simulink model "GridN3"  (R2021a)
settings: Solver=FixedStepAuto  StartTime=0  StopTime=0.2  FixedStep=0.2  RelTol=1e-3
libraries: spsDistributedParametersLineLib x23, spsThreePhaseSeriesRLCLoadLib x6, spsThreePhaseVIMeasurementLib x2, spsGroundLib x1, spsThreePhaseSourceLib x1, spsSeriesRLCBranchLib x1, spspowerguiLib x1
settings Model: Creator=miair  LastModifiedBy=Admin
settings SolverCC: AlgebraicLoopSolver=TrustRegion
settings DebuggingCC: SFMachineParentedDataDiag=warning  ArithmeticOperatorsInVariantConditions=warning
settings SFSimCC: SimUseLocalCustomCode=off  CustomCodeUndefinedFunction=UseInterfaceOnly
settings RTWCC: RTWUseLocalCustomCode=off
settings CodeAppCC: StateflowObjectComments=on
settings SimscapeCC: SimscapeNormalizeSystem=off

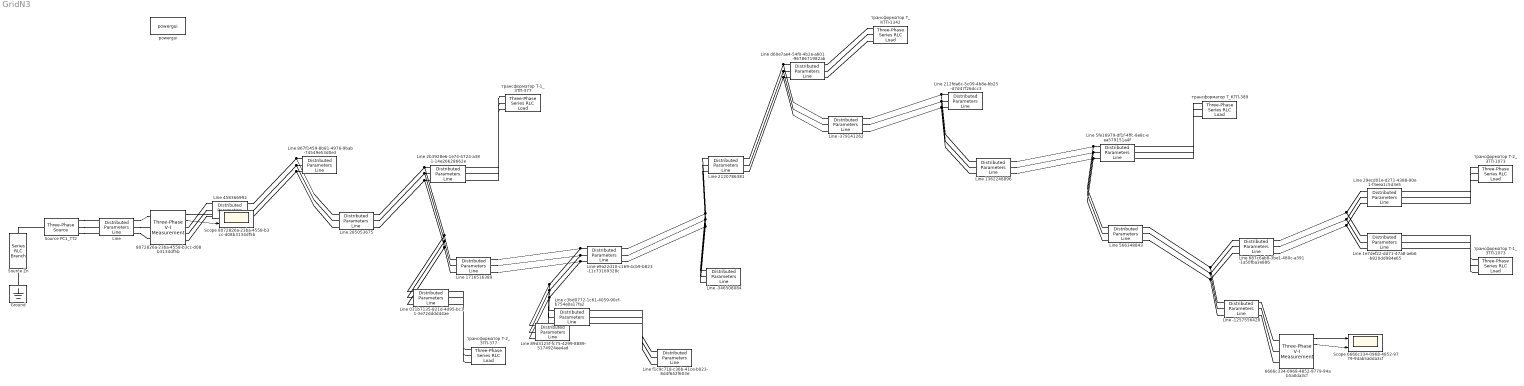
== system GridN3 ==
  6666c334-0968-4852-9779-94ab5a0da3cf : spsThreePhaseVIMeasurementLib/Three-Phase V-I Measurement  VoltageMeasurement=phase-to-ground  SetLabelV=off  LabelV=Vabc  Vpu=off  VpuLL=off  CurrentMeasurement=yes  SetLabelI=off  LabelI=Iabc  Ipu=off  Pbase=100e6  Vbase=500e3  OutputType=Complex  PhasorSimulation=on  PSBequivalent=0
  8072826a-23ba-4558-b3cc-d08b3134df5b : spsThreePhaseVIMeasurementLib/Three-Phase V-I Measurement  VoltageMeasurement=phase-to-ground  SetLabelV=off  LabelV=Vabc  Vpu=off  VpuLL=off  CurrentMeasurement=yes  SetLabelI=off  LabelI=Iabc  Ipu=off  Pbase=100e6  Vbase=500e3  OutputType=Complex  PhasorSimulation=on  PSBequivalent=0
  Ground : spsGroundLib/Ground  LConnTagsString=a
  Line : spsDistributedParametersLineLib/Distributed Parameters Line  Phases=3  Length=0.01  Frequency=50  Resistance=[0.476003738225748 0.351747138225748 0.351747138225748;0.351747138225748 0.476003738225748 0.351747138225748;0.351747138225748 0.351747138225748 0.476003738225748]  Inductance=[0.000705954362986426 0.000459934243504405 0.000459934243504405;0.000459934243504405 0.000705954362986426 0.000459934243504405;0.000459934243504405 0.000459934243504405 0.000705954362986426]  Capacitance=[5.7561313269996e-07 -1.37543883484145e-07 -1.37543912800485e-07;-1.37543883484145e-07 5.75613027339387e-07 -1.37543875208088e-07;-1.37543912800485e-07 -1.37543875208088e-07 5.75613005057695e-07]  x1=[0.00248416968645642 9994.62949178778 9994.63015557589;314.159265358979 314.159265358979 314.159265358979;-0.209307472059049 -0.0974986098841589 -1.66829496511214]  x2=[0.00249202348785049 9994.60556041834 9994.60622450589;314.159265358979 314.159265358979 314.159265358979;-0.209371282448909 -0.0974995948061754 -1.66829595013455]  x3=[0.000641970470002415 520.655471222364 520.655272877081;314.159265358979 314.159265358979 314.159265358979;-0.616333515223182 -0.0919011652667847 -1.6626988448985]  x4=[0.00058046578213103 555.532346643067 555.53252577177;314.159265358979 314.159265358979 314.159265358979;2.4791127944815 -0.102785899279316 -1.6735810096435]  x5=2.2104317621921e-07  V1=[9.635 6853 6854;314.2 314.2 314.2;-1.242 -0.5939 -2.165]  V2=[9.699 6846 6847;314.2 314.2 314.2;-1.252 -0.5942 -2.166]  I1=[9.527 4746 4750;314.2 314.2 314.2;-2.657 2.284 0.7135]  I2=[9.488 5462 5466;314.2 314.2 314.2;0.457 -0.8227 -2.393]  nHarmo=1  Measurements=None  Decoupling=off  VsMag0=0  VrMag0=0  VsAngle0=0  VrAngle0=0  IsMag0=0  IrMag0=0  IsAngle0=0  IrAngle0=0
      settings: SourceProductBaseCode=PS
  Line -1257556428 : spsDistributedParametersLineLib/Distributed Parameters Line  Description=Line connected to devices: [Опора-7/3_РВА-18-10кВ, ВВ РВА-19-10кВ]  Phases=3  Length=0.083645  Frequency=50  Resistance=[0.646656091154803 0.0486237908083191 0.0486712220507153;0.0486237908083191 0.646561225344642 0.0486237934466192;0.0486712220507153 0.0486237934466192 0.646656091154803]  Inductance=[0.00282448912315926 0.00133270803418135 0.00132951476746136;0.00133270803418135 0.00282479813276775 0.00133799988507366;0.00132951476746136 0.00133799988507366 0.00282448912315926]  Capacitance=[7.89543174552926e-09 -1.85986777702161e-09 -1.7901190036642e-09;-1.85986777702161e-09 7.82540023894543e-09 -1.8957321828871e-09;-1.7901190036642e-09 -1.8957321828871e-09 7.91264394645417e-09]  x1=[130.195487453536 9973.60649370411 9972.72701785655;314.159265358979 314.159265358979 314.159265358979;1.01783084349048 -0.180232565928728 -1.7511791412125]  x2=[130.195488485517 9973.60654359898 9972.72706784203;314.159265358979 314.159265358979 314.159265358979;1.01783084007243 -0.180232572293712 -1.75117914763134]  x3=[0.1138298319704 25.37931125459 25.5719653581981;314.159265358979 314.159265358979 314.159265358979;1.01770493460482 -0.180332596029893 -1.75127926654323]  x4=[0.113829831668174 25.3793112552595 25.5719653590152;314.159265358979 314.159265358979 314.159265358979;1.01783083789995 -0.180232572291638 -1.75117914764327]  x5=4.00782735046359e-07  V1=ones(3,3)  V2=ones(3,3)  I1=ones(3,3)  I2=ones(3,3)  nHarmo=1  Measurements=None  Decoupling=off  VsMag0=0  VrMag0=0  VsAngle0=0  VrAngle0=0  IsMag0=0  IrMag0=0  IsAngle0=0  IrAngle0=0
      settings: SourceProductBaseCode=PS
  Line -346508084 : spsDistributedParametersLineLib/Distributed Parameters Line  Description=Line connected to devices: [Опора-2/18_РВА-18-10кВ, трансформатор Т_ТП-1060]  Phases=3  Length=0.088705  Frequency=50  Resistance=[0.991907494602668 0.595664141602668 0.595664141602668;0.595664141602668 0.991907494602668 0.595664141602668;0.595664141602668 0.595664141602668 0.991907494602668]  Inductance=[0.0013307605340619 0.0010400448682494 0.0010400448682494;0.0010400448682494 0.0013307605340619 0.0010400448682494;0.0010400448682494 0.0010400448682494 0.0013307605340619]  Capacitance=[4.05772665830295e-07 -7.83285059789075e-08 -7.83285016498931e-08;-7.83285059789075e-08 4.05772632089447e-07 -7.83285164513028e-08;-7.83285016498931e-08 -7.83285164513028e-08 4.05772808751434e-07]  x1=[0.322741475387784 9980.65599219644 9980.715327366;314.159265358979 314.159265358979 314.159265358979;1.57918467580644 -2.60997141443051 2.10241712331379]  x2=[0.322741581891787 9980.65653761441 9980.71587278735;314.159265358979 314.159265358979 314.159265358979;1.57918400360962 -2.60997165152103 2.10241688622321]  x3=[0.00275476842510044 406.842013048205 406.844478176611;314.159265358979 314.159265358979 314.159265358979;1.57837201879215 -2.61030213099678 2.10208640670926]  x4=[0.00275476820549943 406.842013056325 406.844478184102;314.159265358979 314.159265358979 314.159265358979;1.57918399796258 -2.60997165152122 2.10241688622338]  x5=2.58571089417873e-06  V1=ones(3,3)  V2=ones(3,3)  I1=ones(3,3)  I2=ones(3,3)  nHarmo=1  Measurements=None  Decoupling=off  VsMag0=0  VrMag0=0  VsAngle0=0  VrAngle0=0  IsMag0=0  IrMag0=0  IsAngle0=0  IrAngle0=0
      settings: SourceProductBaseCode=PS
  Line -379141262 : spsDistributedParametersLineLib/Distributed Parameters Line  Description=Line connected to devices: [Опора-2/22_РВА-18-10кВ, СШ ЗТП-921]  Phases=3  Length=0.22086  Frequency=50  Resistance=[0.646656091154803 0.0486237908083191 0.0486712220507153;0.0486237908083191 0.646561225344642 0.0486237934466192;0.0486712220507153 0.0486237934466192 0.646656091154803]  Inductance=[0.00282448912315926 0.00133270803418135 0.00132951476746136;0.00133270803418135 0.00282479813276775 0.00133799988507366;0.00132951476746136 0.00133799988507366 0.00282448912315926]  Capacitance=[7.89543174552926e-09 -1.85986777702161e-09 -1.7901190036642e-09;-1.85986777702161e-09 7.82540023894543e-09 -1.8957321828871e-09;-1.7901190036642e-09 -1.8957321828871e-09 7.91264394645417e-09]  x1=[130.165118685914 9978.39489936247 9977.50969652403;314.159265358979 314.159265358979 314.159265358979;1.01744582863773 -0.18016998377822 -1.75111864820754]  x2=[130.176001379297 9976.68210649216 9975.79896258531;314.159265358979 314.159265358979 314.159265358979;1.01750951020536 -0.180250877136813 -1.75119885149384]  x3=[0.143503097471827 14.6204712251411 14.807865796718;314.159265358979 314.159265358979 314.159265358979;0.904160202139517 -0.00692122857702061 -1.58029304999096]  x4=[0.0865457133359061 36.4569106401023 36.6508234353249;314.159265358979 314.159265358979 314.159265358979;1.20564086316834 -0.249597634104575 -1.82009652208986]  x5=1.0582446633073e-06  V1=ones(3,3)  V2=ones(3,3)  I1=ones(3,3)  I2=ones(3,3)  nHarmo=1  Measurements=None  Decoupling=off  VsMag0=0  VrMag0=0  VsAngle0=0  VrAngle0=0  IsMag0=0  IrMag0=0  IsAngle0=0  IrAngle0=0
      settings: SourceProductBaseCode=PS
  Line 011b7135-821d-4d95-bc11-3e72dddd44ae : spsDistributedParametersLineLib/Distributed Parameters Line  Description=Line connected to devices: [СШ ЗТП-377, трансформатор Т-2_ЗТП-377]  Phases=3  Length=0.005  Frequency=50  Resistance=[0.476003738225748 0.351747138225748 0.351747138225748;0.351747138225748 0.476003738225748 0.351747138225748;0.351747138225748 0.351747138225748 0.476003738225748]  Inductance=[0.000705954362986426 0.000459934243504405 0.000459934243504405;0.000459934243504405 0.000705954362986426 0.000459934243504405;0.000459934243504405 0.000459934243504405 0.000705954362986426]  Capacitance=[5.7561313269996e-07 -1.37543883484145e-07 -1.37543912800485e-07;-1.37543883484145e-07 5.75613027339387e-07 -1.37543875208088e-07;-1.37543912800485e-07 -1.37543875208088e-07 5.75613005057695e-07]  x1=[0.17773558904682 9986.83524772418 9986.84777240376;314.159265358979 314.159265358979 314.159265358979;1.57387195605158 -0.0979022858615706 -1.66869551778252]  x2=[0.177735589236644 9986.83328033485 9986.84580501196;314.159265358979 314.159265358979 314.159265358979;1.5738719572252 -0.0979023740770764 -1.66869560599802]  x3=[0.00241634836079757 534.761421541469 534.762050619376;314.159265358979 314.159265358979 314.159265358979;1.57386230357859 -0.0971689086451658 -1.6679621404806]  x4=[0.00241626858916983 540.599683029839 540.600319451113;314.159265358979 314.159265358979 314.159265358979;1.57384741414391 -0.0986485249011561 -1.66944175689711]  x5=1.10521588109605e-07  V1=ones(3,3)  V2=ones(3,3)  I1=ones(3,3)  I2=ones(3,3)  nHarmo=1  Measurements=None  Decoupling=off  VsMag0=0  VrMag0=0  VsAngle0=0  VrAngle0=0  IsMag0=0  IrMag0=0  IsAngle0=0  IrAngle0=0
      settings: SourceProductBaseCode=PS
  Line 1362246896 : spsDistributedParametersLineLib/Distributed Parameters Line  Description=Line connected to devices: [СШ ЗТП-921, СШ КТП-389]  Phases=3  Length=0.37012  Frequency=50  Resistance=[0.646656091154803 0.0486237908083191 0.0486712220507153;0.0486237908083191 0.646561225344642 0.0486237934466192;0.0486712220507153 0.0486237934466192 0.646656091154803]  Inductance=[0.00282448912315926 0.00133270803418135 0.00132951476746136;0.00133270803418135 0.00282479813276775 0.00133799988507366;0.00132951476746136 0.00133799988507366 0.00282448912315926]  Capacitance=[7.89543174552926e-09 -1.85986777702161e-09 -1.7901190036642e-09;-1.85986777702161e-09 7.82540023894543e-09 -1.8957321828871e-09;-1.7901190036642e-09 -1.8957321828871e-09 7.91264394645417e-09]  x1=[130.176001379297 9976.68210649216 9975.79896258531;314.159265358979 314.159265358979 314.159265358979;1.01728483128456 -0.180429369782926 -1.75137751405231]  x2=[130.194225035775 9973.80842816353 9972.92874137345;314.159265358979 314.159265358979 314.159265358979;1.01739152161977 -0.180564547161652 -1.75151153276431]  x3=[0.143492142355917 14.6158403548629 14.8031186898326;314.159265358979 314.159265358979 314.159265358979;0.904029416141791 -0.00596472151838081 -1.57934691854335]  x4=[0.0865597733675299 36.4458386512353 36.6396270843574;314.159265358979 314.159265358979 314.159265358979;1.20514054087434 -0.250500004942214 -1.8209978227032]  x5=1.77341988039164e-06  V1=ones(3,3)  V2=ones(3,3)  I1=ones(3,3)  I2=ones(3,3)  nHarmo=1  Measurements=None  Decoupling=off  VsMag0=0  VrMag0=0  VsAngle0=0  VrAngle0=0  IsMag0=0  IrMag0=0  IsAngle0=0  IrAngle0=0
      settings: SourceProductBaseCode=PS
  Line 1716516389 : spsDistributedParametersLineLib/Distributed Parameters Line  Description=Line connected to devices: [СШ ЗТП-377, Опора-2/17_РВА-18-10кВ]  Phases=3  Length=0.75608  Frequency=50  Resistance=[0.646656091154803 0.0486237908083191 0.0486712220507153;0.0486237908083191 0.646561225344642 0.0486237934466192;0.0486712220507153 0.0486237934466192 0.646656091154803]  Inductance=[0.00282448912315926 0.00133270803418135 0.00132951476746136;0.00133270803418135 0.00282479813276775 0.00133799988507366;0.00132951476746136 0.00133799988507366 0.00282448912315926]  Capacitance=[7.89543174552926e-09 -1.85986777702161e-09 -1.7901190036642e-09;-1.85986777702161e-09 7.82540023894543e-09 -1.8957321828871e-09;-1.7901190036642e-09 -1.8957321828871e-09 7.91264394645417e-09]  x1=[130.118313913917 9985.79519670877 9984.90187535777;314.159265358979 314.159265358979 314.159265358979;1.01634983279366 -0.18043106645957 -1.75138338253962]  x2=[130.154916249392 9980.00307196193 9979.11599361846;314.159265358979 314.159265358979 314.159265358979;1.01657924988868 -0.180731887694085 -1.75168181382346]  x3=[0.144111783306389 14.4043334623774 14.5925527803305;314.159265358979 314.159265358979 314.159265358979;0.909094978981594 -0.0335791771889403 -1.60667626760913]  x4=[0.0855816272367792 36.5801993239418 36.7739674544058;314.159265358979 314.159265358979 314.159265358979;1.19637429619251 -0.238919524524774 -1.80947527847957]  x5=3.62273668855104e-06  V1=ones(3,3)  V2=ones(3,3)  I1=ones(3,3)  I2=ones(3,3)  nHarmo=1  Measurements=None  Decoupling=off  VsMag0=0  VrMag0=0  VsAngle0=0  VrAngle0=0  IsMag0=0  IrMag0=0  IsAngle0=0  IrAngle0=0
      settings: SourceProductBaseCode=PS
  Line 1e7def22-dd71-47a8-aeb6-b820dd984e65 : spsDistributedParametersLineLib/Distributed Parameters Line  Description=Line connected to devices: [СШ ЗТП-1073, трансформатор Т-1_ЗТП-1073]  Phases=3  Length=0.005  Frequency=50  Resistance=[0.476003738225748 0.351747138225748 0.351747138225748;0.351747138225748 0.476003738225748 0.351747138225748;0.351747138225748 0.351747138225748 0.476003738225748]  Inductance=[0.000705954362986426 0.000459934243504405 0.000459934243504405;0.000459934243504405 0.000705954362986426 0.000459934243504405;0.000459934243504405 0.000459934243504405 0.000705954362986426]  Capacitance=[5.7561313269996e-07 -1.37543883484145e-07 -1.37543912800485e-07;-1.37543883484145e-07 5.75613027339387e-07 -1.37543875208088e-07;-1.37543912800485e-07 -1.37543875208088e-07 5.75613005057695e-07]  x1=[0.451812690641645 9974.47220870287 9974.50474720348;314.159265358979 314.159265358979 314.159265358979;1.55913057537156 -0.0985075295912872 -1.66929601137785]  x2=[0.451812691085289 9974.46940884667 9974.50194733812;314.159265358979 314.159265358979 314.159265358979;1.55913057541318 -0.0985076293003363 -1.6692961110869]  x3=[0.00614243825291168 533.048287175426 533.049984532814;314.159265358979 314.159265358979 314.159265358979;1.55910910621463 -0.0968916516643738 -1.66768013325113]  x4=[0.00614231000061788 540.982652430489 540.984375724773;314.159265358979 314.159265358979 314.159265358979;1.55911722401662 -0.100120461107617 -1.67090894308074]  x5=1.10521588109605e-07  V1=ones(3,3)  V2=ones(3,3)  I1=ones(3,3)  I2=ones(3,3)  nHarmo=1  Measurements=None  Decoupling=off  VsMag0=0  VrMag0=0  VsAngle0=0  VrAngle0=0  IsMag0=0  IrMag0=0  IsAngle0=0  IrAngle0=0
      settings: SourceProductBaseCode=PS
  Line 2120786381 : spsDistributedParametersLineLib/Distributed Parameters Line  Description=Line connected to devices: [Опора-2/18_РВА-18-10кВ, Опора-2/22_РВА-18-10кВ]  Phases=3  Length=0.1588  Frequency=50  Resistance=[0.646656091154803 0.0486237908083191 0.0486712220507153;0.0486237908083191 0.646561225344642 0.0486237934466192;0.0486712220507153 0.0486237934466192 0.646656091154803]  Inductance=[0.00282448912315926 0.00133270803418135 0.00132951476746136;0.00133270803418135 0.00282479813276775 0.00133799988507366;0.00132951476746136 0.00133799988507366 0.00282448912315926]  Capacitance=[7.89543174552926e-09 -1.85986777702161e-09 -1.7901190036642e-09;-1.85986777702161e-09 7.82540023894543e-09 -1.8957321828871e-09;-1.7901190036642e-09 -1.8957321828871e-09 7.91264394645417e-09]  x1=[130.157233586626 9979.63707308602 9978.75041022749;314.159265358979 314.159265358979 314.159265358979;1.01749240903732 -0.180035825758563 -1.75098492254884]  x2=[130.165118685914 9978.39489936247 9977.50969652403;314.159265358979 314.159265358979 314.159265358979;1.0175392466588 -0.180095769295989 -1.75104436307838]  x3=[0.143997402904726 14.4560207631459 14.6435196074342;314.159265358979 314.159265358979 314.159265358979;0.9045960542434 -0.00906035147968803 -1.58243777345835]  x4=[0.0860493978003394 36.6196778627995 36.8136783671172;314.159265358979 314.159265358979 314.159265358979;1.20689131079091 -0.247426152237694 -1.81793500997865]  x5=7.6088586676265e-07  V1=ones(3,3)  V2=ones(3,3)  I1=ones(3,3)  I2=ones(3,3)  nHarmo=1  Measurements=None  Decoupling=off  VsMag0=0  VrMag0=0  VsAngle0=0  VrAngle0=0  IsMag0=0  IrMag0=0  IsAngle0=0  IrAngle0=0
      settings: SourceProductBaseCode=PS
  Line 212fda6c-5c09-4b8e-bb25-d7d47f26dcc3 : spsDistributedParametersLineLib/Distributed Parameters Line  Description=Line connected to devices: [СШ ЗТП-921, разъединитель ЗТП-921]  Phases=3  Length=0.005  Frequency=50  Resistance=[0.476003738225748 0.351747138225748 0.351747138225748;0.351747138225748 0.476003738225748 0.351747138225748;0.351747138225748 0.351747138225748 0.476003738225748]  Inductance=[0.000705954362986426 0.000459934243504405 0.000459934243504405;0.000459934243504405 0.000705954362986426 0.000459934243504405;0.000459934243504405 0.000459934243504405 0.000705954362986426]  Capacitance=[5.7561313269996e-07 -1.37543883484145e-07 -1.37543912800485e-07;-1.37543883484145e-07 5.75613027339387e-07 -1.37543875208088e-07;-1.37543912800485e-07 -1.37543875208088e-07 5.75613005057695e-07]  x1=[0.383357448150149 9977.71827736987 9977.74561261238;314.159265358979 314.159265358979 314.159265358979;1.56396199021545 -0.0983620788695469 -1.66915174413939]  x2=[0.383357448376427 9977.71827952959 9977.7456147721;314.159265358979 314.159265358979 314.159265358979;1.56396198889324 -0.0983620792175357 -1.66915174448738]  x3=[0.00521172839279426 537.18961032381 537.191040498326;314.159265358979 314.159265358979 314.159265358979;1.56392804510435 -0.0983828854951205 -1.66917255074413]  x4=[0.00521172693409196 537.189610335121 537.191040503979;314.159265358979 314.159265358979 314.159265358979;1.56396097637105 -0.0983620792052229 -1.66915174449363]  x5=1.10521588109605e-07  V1=ones(3,3)  V2=ones(3,3)  I1=ones(3,3)  I2=ones(3,3)  nHarmo=1  Measurements=None  Decoupling=off  VsMag0=0  VrMag0=0  VsAngle0=0  VrAngle0=0  IsMag0=0  IrMag0=0  IsAngle0=0  IrAngle0=0
      settings: SourceProductBaseCode=PS
  Line 285053675 : spsDistributedParametersLineLib/Distributed Parameters Line  Description=Line connected to devices: [Опора-1/6_РВА-18-10кВ, СШ ЗТП-377]  Phases=3  Length=0.38821  Frequency=50  Resistance=[0.646656091154803 0.0486237908083191 0.0486712220507153;0.0486237908083191 0.646561225344642 0.0486237934466192;0.0486712220507153 0.0486237934466192 0.646656091154803]  Inductance=[0.00282448912315926 0.00133270803418135 0.00132951476746136;0.00133270803418135 0.00282479813276775 0.00133799988507366;0.00132951476746136 0.00133799988507366 0.00282448912315926]  Capacitance=[7.89543174552926e-09 -1.85986777702161e-09 -1.7901190036642e-09;-1.85986777702161e-09 7.82540023894543e-09 -1.8957321828871e-09;-1.7901190036642e-09 -1.8957321828871e-09 7.91264394645417e-09]  x1=[130.089554391914 9990.38138587262 9989.48346812031;314.159265358979 314.159265358979 314.159265358979;1.01671521116563 -0.179741102610176 -1.75069492136332]  x2=[130.118313913917 9985.79519670877 9984.90187535778;314.159265358979 314.159265358979 314.159265358979;1.01690358218797 -0.179991148934945 -1.75094304624466]  x3=[0.1619203854806 8.5023137742262 8.67905507496919;314.159265358979 314.159265358979 314.159265358979;0.874345194372759 0.173842138150448 -1.40526078541249]  x4=[0.0709888901583562 42.9406072191942 43.135287067239;314.159265358979 314.159265358979 314.159265358979;1.34561825050758 -0.248778960620455 -1.81930098842366]  x5=1.86009762176277e-06  V1=ones(3,3)  V2=ones(3,3)  I1=ones(3,3)  I2=ones(3,3)  nHarmo=1  Measurements=None  Decoupling=off  VsMag0=0  VrMag0=0  VsAngle0=0  VrAngle0=0  IsMag0=0  IrMag0=0  IsAngle0=0  IrAngle0=0
      settings: SourceProductBaseCode=PS
  Line 29ecd01e-d271-4388-90e1-f3eea1c5d3e5 : spsDistributedParametersLineLib/Distributed Parameters Line  Description=Line connected to devices: [СШ ЗТП-1073, трансформатор Т-2_ЗТП-1073]  Phases=3  Length=0.005  Frequency=50  Resistance=[0.476003738225748 0.351747138225748 0.351747138225748;0.351747138225748 0.476003738225748 0.351747138225748;0.351747138225748 0.351747138225748 0.476003738225748]  Inductance=[0.000705954362986426 0.000459934243504405 0.000459934243504405;0.000459934243504405 0.000705954362986426 0.000459934243504405;0.000459934243504405 0.000459934243504405 0.000705954362986426]  Capacitance=[5.7561313269996e-07 -1.37543883484145e-07 -1.37543912800485e-07;-1.37543883484145e-07 5.75613027339387e-07 -1.37543875208088e-07;-1.37543912800485e-07 -1.37543875208088e-07 5.75613005057695e-07]  x1=[0.451812690641645 9974.47220870287 9974.50474720348;314.159265358979 314.159265358979 314.159265358979;1.55913057537156 -0.0985075295912872 -1.66929601137785]  x2=[0.45181269102108 9974.47028696593 9974.50282546024;314.159265358979 314.159265358979 314.159265358979;1.55913057499682 -0.0985076093930357 -1.6692960911796]  x3=[0.00614241735748807 534.210210829071 534.211911945213;314.159265358979 314.159265358979 314.159265358979;1.55910522055333 -0.0976503866358389 -1.66843886833601]  x4=[0.00614233064758624 539.819776519497 539.821496051699;314.159265358979 314.159265358979 314.159265358979;1.55912082453343 -0.0993765433971049 -1.67016502525528]  x5=1.10521588109605e-07  V1=ones(3,3)  V2=ones(3,3)  I1=ones(3,3)  I2=ones(3,3)  nHarmo=1  Measurements=None  Decoupling=off  VsMag0=0  VrMag0=0  VsAngle0=0  VrAngle0=0  IsMag0=0  IrMag0=0  IsAngle0=0  IrAngle0=0
      settings: SourceProductBaseCode=PS
  Line 2b3928e6-1e74-4724-a381-14e26628662e : spsDistributedParametersLineLib/Distributed Parameters Line  Description=Line connected to devices: [СШ ЗТП-377, трансформатор Т-1_ЗТП-377]  Phases=3  Length=0.005  Frequency=50  Resistance=[0.476003738225748 0.351747138225748 0.351747138225748;0.351747138225748 0.476003738225748 0.351747138225748;0.351747138225748 0.351747138225748 0.476003738225748]  Inductance=[0.000705954362986426 0.000459934243504405 0.000459934243504405;0.000459934243504405 0.000705954362986426 0.000459934243504405;0.000459934243504405 0.000459934243504405 0.000705954362986426]  Capacitance=[5.7561313269996e-07 -1.37543883484145e-07 -1.37543912800485e-07;-1.37543883484145e-07 5.75613027339387e-07 -1.37543875208088e-07;-1.37543912800485e-07 -1.37543875208088e-07 5.75613005057695e-07]  x1=[0.17773558904682 9986.83524772418 9986.84777240376;314.159265358979 314.159265358979 314.159265358979;1.57387195605158 -0.0979022858615706 -1.66869551778252]  x2=[0.177735589257299 9986.83297479271 9986.84549946943;314.159265358979 314.159265358979 314.159265358979;1.57387195757025 -0.0979023881020675 -1.66869562002302]  x3=[0.00241635428456539 534.305767182708 534.306395692993;314.159265358979 314.159265358979 314.159265358979;1.57386549740141 -0.0970597102712424 -1.66785294212386]  x4=[0.00241626159216721 541.055413034098 541.056050022876;314.159265358979 314.159265358979 314.159265358979;1.57384448596031 -0.0987551287904001 -1.66954836077086]  x5=1.10521588109605e-07  V1=ones(3,3)  V2=ones(3,3)  I1=ones(3,3)  I2=ones(3,3)  nHarmo=1  Measurements=None  Decoupling=off  VsMag0=0  VrMag0=0  VsAngle0=0  VrAngle0=0  IsMag0=0  IrMag0=0  IsAngle0=0  IrAngle0=0
      settings: SourceProductBaseCode=PS
  Line 458366992 : spsDistributedParametersLineLib/Distributed Parameters Line  Description=Line connected to devices: [ВВ РВА-18-10кВ, Опора-1/6_РВА-18-10кВ]  Phases=3  Length=0.26932  Frequency=50  Resistance=[0.646656091154803 0.0486237908083191 0.0486712220507153;0.0486237908083191 0.646561225344642 0.0486237934466192;0.0486712220507153 0.0486237934466192 0.646656091154803]  Inductance=[0.00282448912315926 0.00133270803418135 0.00132951476746136;0.00133270803418135 0.00282479813276775 0.00133799988507366;0.00132951476746136 0.00133799988507366 0.00282448912315926]  Capacitance=[7.89543174552926e-09 -1.85986777702161e-09 -1.7901190036642e-09;-1.85986777702161e-09 7.82540023894543e-09 -1.8957321828871e-09;-1.7901190036642e-09 -1.8957321828871e-09 7.91264394645417e-09]  x1=[130.06957908201 9993.56214605898 9992.66103161426;314.159265358979 314.159265358979 314.159265358979;1.01676353023063 -0.179425432203557 -1.75038044609108]  x2=[130.089554391913 9990.38138587262 9989.48346812031;314.159265358979 314.159265358979 314.159265358979;1.01689417456436 -0.179598927943846 -1.75055261135677]  x3=[0.161920197488385 8.51044085838394 8.68730204071955;314.159265358979 314.159265358979 314.159265358979;0.874137414852068 0.173189764757969 -1.40590036844201]  x4=[0.0709845073730207 42.9560301669031 43.150853235089;314.159265358979 314.159265358979 314.159265358979;1.34650369715478 -0.248194219071961 -1.81871576123058]  x5=1.29043943096043e-06  V1=ones(3,3)  V2=ones(3,3)  I1=ones(3,3)  I2=ones(3,3)  nHarmo=1  Measurements=None  Decoupling=off  VsMag0=0  VrMag0=0  VsAngle0=0  VrAngle0=0  IsMag0=0  IrMag0=0  IsAngle0=0  IrAngle0=0
      settings: SourceProductBaseCode=PS
  Line 566348843 : spsDistributedParametersLineLib/Distributed Parameters Line  Description=Line connected to devices: [СШ КТП-389, Опора-7/3_РВА-18-10кВ]  Phases=3  Length=0.043512  Frequency=50  Resistance=[0.646656091154803 0.0486237908083191 0.0486712220507153;0.0486237908083191 0.646561225344642 0.0486237934466192;0.0486712220507153 0.0486237934466192 0.646656091154803]  Inductance=[0.00282448912315926 0.00133270803418135 0.00132951476746136;0.00133270803418135 0.00282479813276775 0.00133799988507366;0.00132951476746136 0.00133799988507366 0.00282448912315926]  Capacitance=[7.89543174552926e-09 -1.85986777702161e-09 -1.7901190036642e-09;-1.85986777702161e-09 7.82540023894543e-09 -1.8957321828871e-09;-1.7901190036642e-09 -1.8957321828871e-09 7.91264394645417e-09]  x1=[130.194225035775 9973.80842816353 9972.92874137345;314.159265358979 314.159265358979 314.159265358979;1.01788315992183 -0.180173972820492 -1.75112058662403]  x2=[130.195487453537 9973.60649370411 9972.72701785656;314.159265358979 314.159265358979 314.159265358979;1.01789125511535 -0.180184572860482 -1.75113110245825]  x3=[0.132135084964361 18.6509537392264 18.8419614076192;314.159265358979 314.159265358979 314.159265358979;0.948982193224668 -0.112644177350074 -1.68437306389605]  x4=[0.096271591376695 32.1777012824909 32.3712689228071;314.159265358979 314.159265358979 314.159265358979;1.1124496063731 -0.219345511337796 -1.79000193534067]  x5=2.08486560671136e-07  V1=ones(3,3)  V2=ones(3,3)  I1=ones(3,3)  I2=ones(3,3)  nHarmo=1  Measurements=None  Decoupling=off  VsMag0=0  VrMag0=0  VsAngle0=0  VrAngle0=0  IsMag0=0  IrMag0=0  IsAngle0=0  IrAngle0=0
      settings: SourceProductBaseCode=PS
  Line 5fe16979-df1f-4ffc-8e8c-eea579151a4f : spsDistributedParametersLineLib/Distributed Parameters Line  Description=Line connected to devices: [СШ КТП-389, трансформатор Т_КТП-389]  Phases=3  Length=0.005  Frequency=50  Resistance=[0.476003738225748 0.351747138225748 0.351747138225748;0.351747138225748 0.476003738225748 0.351747138225748;0.351747138225748 0.351747138225748 0.476003738225748]  Inductance=[0.000705954362986426 0.000459934243504405 0.000459934243504405;0.000459934243504405 0.000705954362986426 0.000459934243504405;0.000459934243504405 0.000459934243504405 0.000705954362986426]  Capacitance=[5.7561313269996e-07 -1.37543883484145e-07 -1.37543912800485e-07;-1.37543883484145e-07 5.75613027339387e-07 -1.37543875208088e-07;-1.37543912800485e-07 -1.37543875208088e-07 5.75613005057695e-07]  x1=[0.447225520649454 9974.84338976336 9974.8756130052;314.159265358979 314.159265358979 314.159265358979;1.55898887476454 -0.0984972350097678 -1.66928579752801]  x2=[0.447225521125626 9974.84027093679 9974.87249416855;314.159265358979 314.159265358979 314.159265358979;1.55898887484724 -0.0984973177377232 -1.66928588025596]  x3=[0.00608008125712268 532.82120306012 532.822882787385;314.159265358979 314.159265358979 314.159265358979;1.55896754611922 -0.0960796723066996 -1.66686823462397]  x4=[0.0060799405236352 541.251404434506 541.253111416591;314.159265358979 314.159265358979 314.159265358979;1.55897542643501 -0.100897869822195 -1.67168643253053]  x5=1.10521588109605e-07  V1=ones(3,3)  V2=ones(3,3)  I1=ones(3,3)  I2=ones(3,3)  nHarmo=1  Measurements=None  Decoupling=off  VsMag0=0  VrMag0=0  VsAngle0=0  VrAngle0=0  IsMag0=0  IrMag0=0  IsAngle0=0  IrAngle0=0
      settings: SourceProductBaseCode=PS
  Line 687c6ab8-3be1-480c-a391-1a50fba3e886 : spsDistributedParametersLineLib/Distributed Parameters Line  Description=Line connected to devices: [Опора-7/3_РВА-18-10кВ, СШ ЗТП-1073]  Phases=3  Length=0.043769  Frequency=50  Resistance=[1.20319872737733 0.650615891377333 0.650615891377333;0.650615891377333 1.20319872737733 0.650615891377333;0.650615891377333 0.650615891377333 1.20319872737733]  Inductance=[0.00152224047491712 0.00121971605345402 0.00121971605345402;0.00121971605345402 0.00152224047491712 0.00121971605345402;0.00121971605345402 0.00121971605345402 0.00152224047491712]  Capacitance=[3.5492678521701e-07 -6.81668751215391e-08 -6.81669173453455e-08;-6.81668751215391e-08 3.54926826597295e-07 -6.81668989311185e-08;-6.81669173453455e-08 -6.81668989311185e-08 3.5492692272688e-07]  x1=[0.454296608443964 9974.61529933371 9974.69997611312;314.159265358979 314.159265358979 314.159265358979;1.56953337458952 0.509936554149113 2.08073253660531]  x2=[0.454296657135368 9974.44614019598 9974.53081553971;314.159265358979 314.159265358979 314.159265358979;1.56953299856961 0.509936858373028 2.08073284082919]  x3=[0.00337224534769466 366.001895291915 366.005056055195;314.159265358979 314.159265358979 314.159265358979;1.56890807612545 0.513380948422595 2.0841769303125]  x4=[0.00337277461754321 379.533930602969 379.537206216854;314.159265358979 314.159265358979 314.159265358979;1.56975350173008 0.506462439448261 2.0772584224104]  x5=1.28802439821471e-06  V1=ones(3,3)  V2=ones(3,3)  I1=ones(3,3)  I2=ones(3,3)  nHarmo=1  Measurements=None  Decoupling=off  VsMag0=0  VrMag0=0  VsAngle0=0  VrAngle0=0  IsMag0=0  IrMag0=0  IsAngle0=0  IrAngle0=0
      settings: SourceProductBaseCode=PS
  Line 867f1459-8b81-4976-9bab-74549e53d0e3 : spsDistributedParametersLineLib/Distributed Parameters Line  Description=Line connected to devices: [Опора-1/6_РВА-18-10кВ, трансформатор КТП-881]  Phases=3  Length=0.00065343  Frequency=50  Resistance=[0.646656091154803 0.0486237908083191 0.0486712220507153;0.0486237908083191 0.646561225344642 0.0486237934466192;0.0486712220507153 0.0486237934466192 0.646656091154803]  Inductance=[0.00282448912315926 0.00133270803418135 0.00132951476746136;0.00133270803418135 0.00282479813276775 0.00133799988507366;0.00132951476746136 0.00133799988507366 0.00282448912315926]  Capacitance=[7.89543174552926e-09 -1.85986777702161e-09 -1.7901190036642e-09;-1.85986777702161e-09 7.82540023894543e-09 -1.8957321828871e-09;-1.7901190036642e-09 -1.8957321828871e-09 7.91264394645417e-09]  x1=[130.089554391914 9990.38138587261 9989.48346812031;314.159265358979 314.159265358979 314.159265358979;1.01729859446924 -0.179277642890909 -1.75023102046322]  x2=[130.08955439198 9990.38138587566 9989.48346812337;314.159265358979 314.159265358979 314.159265358979;1.01729859446904 -0.179277642891298 -1.75023102046361]  x3=[0.11374180914278 25.4244049611891 25.6173760740397;314.159265358979 314.159265358979 314.159265358979;1.01729758625954 -0.179278424356093 -1.75023180237931]  x4=[0.113741805571951 25.4244049643665 25.6173760701135;314.159265358979 314.159265358979 314.159265358979;1.01729862599899 -0.179277642782097 -1.75023102069132]  x5=3.1308920146015e-09  V1=ones(3,3)  V2=ones(3,3)  I1=ones(3,3)  I2=ones(3,3)  nHarmo=1  Measurements=None  Decoupling=off  VsMag0=0  VrMag0=0  VsAngle0=0  VrAngle0=0  IsMag0=0  IrMag0=0  IsAngle0=0  IrAngle0=0
      settings: SourceProductBaseCode=PS
  Line 89d3125f-fc75-4299-8889-5174924ee4ad : spsDistributedParametersLineLib/Distributed Parameters Line  Description=Line connected to devices: [Опора-2/17_РВА-18-10кВ, трансформатор Т_КТП-1374]  Phases=3  Length=0.0029735  Frequency=50  Resistance=[0.991907494602668 0.595664141602668 0.595664141602668;0.595664141602668 0.991907494602668 0.595664141602668;0.595664141602668 0.595664141602668 0.991907494602668]  Inductance=[0.0013307605340619 0.0010400448682494 0.0010400448682494;0.0010400448682494 0.0013307605340619 0.0010400448682494;0.0010400448682494 0.0010400448682494 0.0013307605340619]  Capacitance=[4.05772665830295e-07 -7.83285059789075e-08 -7.83285016498931e-08;-7.83285059789075e-08 4.05772632089447e-07 -7.83285164513028e-08;-7.83285016498931e-08 -7.83285164513028e-08 4.05772808751434e-07]  x1=[0.314513605651154 9981.02261486018 9981.08041260805;314.159265358979 314.159265358979 314.159265358979;1.58076041127244 -2.60963378353415 2.10275476804925]  x2=[0.314513605763482 9981.02261547307 9981.08041322094;314.159265358979 314.159265358979 314.159265358979;1.58076041054879 -2.60963378380057 2.10275476778284]  x3=[0.00268775922794191 407.280128238823 407.282533248584;314.159265358979 314.159265358979 314.159265358979;1.58073410902569 -2.60964486573257 2.10274368587232]  x4=[0.0026877610540507 407.280128244187 407.282533250155;314.159265358979 314.159265358979 314.159265358979;1.58076012427042 -2.60963378378322 2.10275476777234]  x5=8.66761889841661e-08  V1=ones(3,3)  V2=ones(3,3)  I1=ones(3,3)  I2=ones(3,3)  nHarmo=1  Measurements=None  Decoupling=off  VsMag0=0  VrMag0=0  VsAngle0=0  VrAngle0=0  IsMag0=0  IrMag0=0  IsAngle0=0  IrAngle0=0
      settings: SourceProductBaseCode=PS
  Line c3bd0772-1c61-4059-90cf-b754e0a17fa2 : spsDistributedParametersLineLib/Distributed Parameters Line  Description=Line connected to devices: [Опора-2/17_РВА-18-10кВ, разъединитель ЛР-235-10кВ]  Phases=3  Length=7.7673e-05  Frequency=50  Resistance=[0.646656091154803 0.0486237908083191 0.0486712220507153;0.0486237908083191 0.646561225344642 0.0486237934466192;0.0486712220507153 0.0486237934466192 0.646656091154803]  Inductance=[0.00282448912315926 0.00133270803418135 0.00132951476746136;0.00133270803418135 0.00282479813276775 0.00133799988507366;0.00132951476746136 0.00133799988507366 0.00282448912315926]  Capacitance=[7.89543174552926e-09 -1.85986777702161e-09 -1.7901190036642e-09;-1.85986777702161e-09 7.82540023894543e-09 -1.8957321828871e-09;-1.7901190036642e-09 -1.8957321828871e-09 7.91264394645417e-09]  x1=[130.154916249392 9980.00307196194 9979.11599361847;314.159265358979 314.159265358979 314.159265358979;1.0177172492653 -0.179827821930895 -1.75077688745368]  x2=[130.154916187101 9980.00307893015 9979.11600054343;314.159265358979 314.159265358979 314.159265358979;1.01771724966345 -0.179827822819515 -1.75077688834212]  x3=[0.113957620939003 25.3986996495865 25.5915448662652;314.159265358979 314.159265358979 314.159265358979;1.02240022237839 -0.187346138029325 -1.75823937546859]  x4=[0.113642905062116 25.3987559757396 25.591492927039;314.159265358979 314.159265358979 314.159265358979;1.01302094556198 -0.172309615104072 -1.74331447888282]  x5=3.72168060006646e-10  V1=ones(3,3)  V2=ones(3,3)  I1=ones(3,3)  I2=ones(3,3)  nHarmo=1  Measurements=None  Decoupling=off  VsMag0=0  VrMag0=0  VsAngle0=0  VrAngle0=0  IsMag0=0  IrMag0=0  IsAngle0=0  IrAngle0=0
      settings: SourceProductBaseCode=PS
  Line d60e7ae4-54f0-4b2e-a601-9678671982ab : spsDistributedParametersLineLib/Distributed Parameters Line  Description=Line connected to devices: [Опора-2/22_РВА-18-10кВ, трансформатор Т_КТП-1342]  Phases=3  Length=0.088295  Frequency=50  Resistance=[0.991907494602668 0.595664141602668 0.595664141602668;0.595664141602668 0.991907494602668 0.595664141602668;0.595664141602668 0.595664141602668 0.991907494602668]  Inductance=[0.0013307605340619 0.0010400448682494 0.0010400448682494;0.0010400448682494 0.0013307605340619 0.0010400448682494;0.0010400448682494 0.0010400448682494 0.0013307605340619]  Capacitance=[4.05772665830295e-07 -7.83285059789075e-08 -7.83285016498931e-08;-7.83285059789075e-08 4.05772632089447e-07 -7.83285164513028e-08;-7.83285016498931e-08 -7.83285164513028e-08 4.05772808751434e-07]  x1=[0.350492589847978 9979.41174279145 9979.47626259251;314.159265358979 314.159265358979 314.159265358979;1.57588059642484 -2.61002955511633 2.10235893013837]  x2=[0.350492701795593 9979.40602911414 9979.47054887839;314.159265358979 314.159265358979 314.159265358979;1.57587992840381 -2.61002964909706 2.10235883615758]  x3=[0.00299164342258576 406.632472228289 406.635147665729;314.159265358979 314.159265358979 314.159265358979;1.57507251548917 -2.61016892979716 2.10221955539885]  x4=[0.00299166818655791 406.953893730315 406.956571245627;314.159265358979 314.159265358979 314.159265358979;1.57587911218161 -2.61021944188925 2.10216904338628]  x5=2.5737595783948e-06  V1=ones(3,3)  V2=ones(3,3)  I1=ones(3,3)  I2=ones(3,3)  nHarmo=1  Measurements=None  Decoupling=off  VsMag0=0  VrMag0=0  VsAngle0=0  VrAngle0=0  IsMag0=0  IrMag0=0  IsAngle0=0  IrAngle0=0
      settings: SourceProductBaseCode=PS
  Line e9a22d10-c169-4cb9-b823-11c73169328c : spsDistributedParametersLineLib/Distributed Parameters Line  Description=Line connected to devices: [Опора-2/17_РВА-18-10кВ, Опора-2/18_РВА-18-10кВ]  Phases=3  Length=0.047179  Frequency=50  Resistance=[0.646656091154803 0.0486237908083191 0.0486712220507153;0.0486237908083191 0.646561225344642 0.0486237934466192;0.0486712220507153 0.0486237934466192 0.646656091154803]  Inductance=[0.00282448912315926 0.00133270803418135 0.00132951476746136;0.00133270803418135 0.00282479813276775 0.00133799988507366;0.00132951476746136 0.00133799988507366 0.00282448912315926]  Capacitance=[7.89543174552926e-09 -1.85986777702161e-09 -1.7901190036642e-09;-1.85986777702161e-09 7.82540023894543e-09 -1.8957321828871e-09;-1.7901190036642e-09 -1.8957321828871e-09 7.91264394645417e-09]  x1=[130.154916249392 9980.00307196193 9979.11599361847;314.159265358979 314.159265358979 314.159265358979;1.01764634831851 -0.179884148076491 -1.75083326721778]  x2=[130.157233586626 9979.63707308602 9978.75041022749;314.159265358979 314.159265358979 314.159265358979;1.0176604305154 -0.179902343729541 -1.75085131345438]  x3=[0.144072115407757 14.4367546623829 14.6246522555924;314.159265358979 314.159265358979 314.159265358979;0.907379493904356 -0.0182080596105747 -1.59147213414623]  x4=[0.0858726638731459 36.6178134777838 36.8119096585864;314.159265358979 314.159265358979 314.159265358979;1.20325945092685 -0.243442952889275 -1.81397043615756]  x5=2.26056891108281e-07  V1=ones(3,3)  V2=ones(3,3)  I1=ones(3,3)  I2=ones(3,3)  nHarmo=1  Measurements=None  Decoupling=off  VsMag0=0  VrMag0=0  VsAngle0=0  VrAngle0=0  IsMag0=0  IrMag0=0  IsAngle0=0  IrAngle0=0
      settings: SourceProductBaseCode=PS
  Line f1c9c718-c36b-41ce-b023-8d4f642f603e : spsDistributedParametersLineLib/Distributed Parameters Line  Description=Line connected to devices: [разъединитель ЛР-235-10кВ, трансформатор Т_КТП-1303]  Phases=3  Length=0.12578  Frequency=50  Resistance=[0.991907494602668 0.595664141602668 0.595664141602668;0.595664141602668 0.991907494602668 0.595664141602668;0.595664141602668 0.595664141602668 0.991907494602668]  Inductance=[0.0013307605340619 0.0010400448682494 0.0010400448682494;0.0010400448682494 0.0013307605340619 0.0010400448682494;0.0010400448682494 0.0010400448682494 0.0013307605340619]  Capacitance=[4.05772665830295e-07 -7.83285059789075e-08 -7.83285016498931e-08;-7.83285059789075e-08 4.05772632089447e-07 -7.83285164513028e-08;-7.83285016498931e-08 -7.83285164513028e-08 4.05772808751434e-07]  x1=[0.314513566206951 9981.02262181064 9981.0804195534;314.159265358979 314.159265358979 314.159265358979;1.57963650804077 -2.61009147661699 2.10229707491837]  x2=[0.314513774835549 9981.02371847121 9981.08151622057;314.159265358979 314.159265358979 314.159265358979;1.57963515643654 -2.61009195331265 2.10229659822261]  x3=[0.00268314743880937 406.674120017418 406.676521376464;314.159265358979 314.159265358979 314.159265358979;1.57848398822146 -2.61056048920664 2.10182806227537]  x4=[0.00268314751821141 406.674120040046 406.676521399045;314.159265358979 314.159265358979 314.159265358979;1.57963515298713 -2.61009195331271 2.10229659822229]  x5=3.66643048610338e-06  V1=ones(3,3)  V2=ones(3,3)  I1=ones(3,3)  I2=ones(3,3)  nHarmo=1  Measurements=None  Decoupling=off  VsMag0=0  VrMag0=0  VsAngle0=0  VrAngle0=0  IsMag0=0  IrMag0=0  IsAngle0=0  IrAngle0=0
      settings: SourceProductBaseCode=PS
  Scope 6666c334-0968-4852-9779-94ab5a0da3cf : Scope  NumInputPorts=2
  Scope 8072826a-23ba-4558-b3cc-d08b3134df5b : Scope  NumInputPorts=2
  Source PC1_TT2 : spsThreePhaseSourceLib/Three-Phase Source  InternalConnection=Yn  VoltagePhases=off  Voltage=10000  PhaseAngle=0  Voltage_phases=[25e3 25e3 25e3]/sqrt(3)  PhaseAngles_phases=[0 -120 +120]  Frequency=50  NonIdealSource=on  SpecifyImpedance=off  Resistance=0.14  Inductance=0.0031831  ShortCircuitLevel=100e6  BaseVoltage=25e3  XRratio=7  BusType=swing  Pref=10e3  Qref=0  Prefabc=[10e3, 10e3, 10e3]  Qrefabc=[0, 0, 0]  Qmin=-inf  Qmax=inf
  Source Zn : spsSeriesRLCBranchLib/Series RLC Branch  LConnTagsString=__new0  RConnTagsString=__new0  BranchType=RL  Resistance=0.001  Inductance=3.1831e-06  SetiL0=off  InitialCurrent=0  Capacitance=0  Setx0=off  InitialVoltage=0  Measurements=None
  powergui : spspowerguiLib/powergui  Priority=1  SimulationMode=Phasor  SampleTime=50e-6  frequency=50  Iterations=50  frequencyindice=50  Pbase=100e6  ErrMax=1e-4  UnitsV=kV  UnitsW=MW  buscounter=0  FunctionMessages=off  echomessages=off  EnableUseOfTLC=off  CurrentSourceSwitches=off  DisableSnubberDevices=off  DisableRonSwitches=off  DisableVfSwitches=off  DisplayEquations=off  AutomaticDiscreteSolvers=off  SolverType=Tustin/Backward Euler (TBE)  Interpol=off  ExternalGateDelay=off  methode=off  Ts=10  x0status=blocks  SPID=off  SwTol=0  HookPort=off  NonlinearTolerance=1e-4  nMaxIteration=100  ContinueOnMaxIteration=off  RestoreLinks=warning  ResistiveCurrentMeasurement=off  Frange=[0:2:500]  Ylog=off  Xlog=on  ShowGrid=off  save=off  variable=ZData  structure=0  ZoomFFT=off  StartTime=0.0  cycles=1  DisplayStyle=1  fundamental=60  FreqAxis=off  MaxFrequency=1000  frequencyindicesteady=1  RmsSteady=1  display=off
  трансформатор Т-1_ЗТП-1073 : spsThreePhaseSeriesRLCLoadLib/Three-Phase Series RLC Load  Description=Device type: [LOAD], in DispatcherName: [трансформатор Т-1_ЗТП-1073]  LConnTagsString=A|B|C  Configuration=Delta  NominalVoltage=10500  Vabc=[1e3 1e3 1e3]  Vabcp=[1e3 1e3 1e3]  NominalFrequency=50  UnbalancedPower=off  ActivePower=45600  InductivePower=14987.995  CapacitivePower=0  Pabc=[10e3 9e3 11e3]  QLabc=[100 90 110]  QCabc=[100 90 110]  Pabcp=[10e3 9e3 11e3]  QLabcp=[100 90 110]  QCabcp=[100 90 110]  Measurements=None  LoadType=constant Z
  трансформатор Т-1_ЗТП-377 : spsThreePhaseSeriesRLCLoadLib/Three-Phase Series RLC Load  Description=Device type: [LOAD], in DispatcherName: [трансформатор Т-1_ЗТП-377]  LConnTagsString=A|B|C  Configuration=Delta  NominalVoltage=10500  Vabc=[1e3 1e3 1e3]  Vabcp=[1e3 1e3 1e3]  NominalFrequency=50  UnbalancedPower=off  ActivePower=53200  InductivePower=17485.994  CapacitivePower=0  Pabc=[10e3 9e3 11e3]  QLabc=[100 90 110]  QCabc=[100 90 110]  Pabcp=[10e3 9e3 11e3]  QLabcp=[100 90 110]  QCabcp=[100 90 110]  Measurements=None  LoadType=constant Z
  трансформатор Т-2_ЗТП-1073 : spsThreePhaseSeriesRLCLoadLib/Three-Phase Series RLC Load  Description=Device type: [LOAD], in DispatcherName: [трансформатор Т-2_ЗТП-1073]  LConnTagsString=A|B|C  Configuration=Delta  NominalVoltage=10500  Vabc=[1e3 1e3 1e3]  Vabcp=[1e3 1e3 1e3]  NominalFrequency=50  UnbalancedPower=off  ActivePower=45600  InductivePower=14987.995  CapacitivePower=0  Pabc=[10e3 9e3 11e3]  QLabc=[100 90 110]  QCabc=[100 90 110]  Pabcp=[10e3 9e3 11e3]  QLabcp=[100 90 110]  QCabcp=[100 90 110]  Measurements=None  LoadType=constant Z
  трансформатор Т-2_ЗТП-377 : spsThreePhaseSeriesRLCLoadLib/Three-Phase Series RLC Load  Description=Device type: [LOAD], in DispatcherName: [трансформатор Т-2_ЗТП-377]  LConnTagsString=A|B|C  Configuration=Delta  NominalVoltage=10500  Vabc=[1e3 1e3 1e3]  Vabcp=[1e3 1e3 1e3]  NominalFrequency=50  UnbalancedPower=off  ActivePower=53200  InductivePower=17485.994  CapacitivePower=0  Pabc=[10e3 9e3 11e3]  QLabc=[100 90 110]  QCabc=[100 90 110]  Pabcp=[10e3 9e3 11e3]  QLabcp=[100 90 110]  QCabcp=[100 90 110]  Measurements=None  LoadType=constant Z
  трансформатор Т_КТП-1342 : spsThreePhaseSeriesRLCLoadLib/Three-Phase Series RLC Load  Description=Device type: [LOAD], in DispatcherName: [трансформатор Т_КТП-1342]  LConnTagsString=A|B|C  Configuration=Delta  NominalVoltage=10500  Vabc=[1e3 1e3 1e3]  Vabcp=[1e3 1e3 1e3]  NominalFrequency=50  UnbalancedPower=off  ActivePower=1995  InductivePower=655.725  CapacitivePower=0  Pabc=[10e3 9e3 11e3]  QLabc=[100 90 110]  QCabc=[100 90 110]  Pabcp=[10e3 9e3 11e3]  QLabcp=[100 90 110]  QCabcp=[100 90 110]  Measurements=None  LoadType=constant Z
  трансформатор Т_КТП-389 : spsThreePhaseSeriesRLCLoadLib/Three-Phase Series RLC Load  Description=Device type: [LOAD], in DispatcherName: [трансформатор Т_КТП-389]  LConnTagsString=A|B|C  Configuration=Delta  NominalVoltage=10500  Vabc=[1e3 1e3 1e3]  Vabcp=[1e3 1e3 1e3]  NominalFrequency=50  UnbalancedPower=off  ActivePower=90972  InductivePower=29901.05  CapacitivePower=0  Pabc=[10e3 9e3 11e3]  QLabc=[100 90 110]  QCabc=[100 90 110]  Pabcp=[10e3 9e3 11e3]  QLabcp=[100 90 110]  QCabcp=[100 90 110]  Measurements=None  LoadType=constant Z
  wires:
  8072826a-23ba-4558-b3cc-d08b3134df5b/1 -> Scope 8072826a-23ba-4558-b3cc-d08b3134df5b/1
  8072826a-23ba-4558-b3cc-d08b3134df5b/2 -> Scope 8072826a-23ba-4558-b3cc-d08b3134df5b/2
  6666c334-0968-4852-9779-94ab5a0da3cf/1 -> Scope 6666c334-0968-4852-9779-94ab5a0da3cf/1
  6666c334-0968-4852-9779-94ab5a0da3cf/2 -> Scope 6666c334-0968-4852-9779-94ab5a0da3cf/2
  connections:
  Ground/LConn1 -- Source Zn/LConn1
  Source Zn/RConn1 -- Source PC1_TT2/LConn1
  Line 2120786381/LConn1 -- Line e9a22d10-c169-4cb9-b823-11c73169328c/RConn1 -- Line -346508084/LConn1
  Line 2120786381/LConn2 -- Line e9a22d10-c169-4cb9-b823-11c73169328c/RConn2 -- Line -346508084/LConn2
  Line 2120786381/LConn3 -- Line e9a22d10-c169-4cb9-b823-11c73169328c/RConn3 -- Line -346508084/LConn3
  трансформатор Т-1_ЗТП-1073/LConn1 -- Line 1e7def22-dd71-47a8-aeb6-b820dd984e65/RConn1
  трансформатор Т-1_ЗТП-1073/LConn2 -- Line 1e7def22-dd71-47a8-aeb6-b820dd984e65/RConn2
  трансформатор Т-1_ЗТП-1073/LConn3 -- Line 1e7def22-dd71-47a8-aeb6-b820dd984e65/RConn3
  трансформатор Т_КТП-1342/LConn1 -- Line d60e7ae4-54f0-4b2e-a601-9678671982ab/RConn1
  трансформатор Т_КТП-1342/LConn2 -- Line d60e7ae4-54f0-4b2e-a601-9678671982ab/RConn2
  трансформатор Т_КТП-1342/LConn3 -- Line d60e7ae4-54f0-4b2e-a601-9678671982ab/RConn3
  трансформатор Т_КТП-389/LConn1 -- Line 5fe16979-df1f-4ffc-8e8c-eea579151a4f/RConn1
  трансформатор Т_КТП-389/LConn2 -- Line 5fe16979-df1f-4ffc-8e8c-eea579151a4f/RConn2
  трансформатор Т_КТП-389/LConn3 -- Line 5fe16979-df1f-4ffc-8e8c-eea579151a4f/RConn3
  Line 1716516389/LConn1 -- Line 2b3928e6-1e74-4724-a381-14e26628662e/LConn1 -- Line 285053675/RConn1 -- Line 011b7135-821d-4d95-bc11-3e72dddd44ae/LConn1
  Line 1716516389/LConn2 -- Line 2b3928e6-1e74-4724-a381-14e26628662e/LConn2 -- Line 285053675/RConn2 -- Line 011b7135-821d-4d95-bc11-3e72dddd44ae/LConn2
  Line 1716516389/LConn3 -- Line 2b3928e6-1e74-4724-a381-14e26628662e/LConn3 -- Line 285053675/RConn3 -- Line 011b7135-821d-4d95-bc11-3e72dddd44ae/LConn3
  Line 212fda6c-5c09-4b8e-bb25-d7d47f26dcc3/LConn1 -- Line 1362246896/LConn1 -- Line -379141262/RConn1
  Line 212fda6c-5c09-4b8e-bb25-d7d47f26dcc3/LConn2 -- Line 1362246896/LConn2 -- Line -379141262/RConn2
  Line 212fda6c-5c09-4b8e-bb25-d7d47f26dcc3/LConn3 -- Line 1362246896/LConn3 -- Line -379141262/RConn3
  Source PC1_TT2/RConn1 -- Line/LConn1
  Source PC1_TT2/RConn2 -- Line/LConn2
  Source PC1_TT2/RConn3 -- Line/LConn3
  6666c334-0968-4852-9779-94ab5a0da3cf/LConn1 -- Line -1257556428/RConn1
  6666c334-0968-4852-9779-94ab5a0da3cf/LConn2 -- Line -1257556428/RConn2
  6666c334-0968-4852-9779-94ab5a0da3cf/LConn3 -- Line -1257556428/RConn3
  Line -1257556428/LConn1 -- Line 687c6ab8-3be1-480c-a391-1a50fba3e886/LConn1 -- Line 566348843/RConn1
  Line -1257556428/LConn2 -- Line 687c6ab8-3be1-480c-a391-1a50fba3e886/LConn2 -- Line 566348843/RConn2
  Line -1257556428/LConn3 -- Line 687c6ab8-3be1-480c-a391-1a50fba3e886/LConn3 -- Line 566348843/RConn3
  Line c3bd0772-1c61-4059-90cf-b754e0a17fa2/LConn1 -- Line e9a22d10-c169-4cb9-b823-11c73169328c/LConn1 -- Line 1716516389/RConn1 -- Line 89d3125f-fc75-4299-8889-5174924ee4ad/LConn1
  Line c3bd0772-1c61-4059-90cf-b754e0a17fa2/LConn2 -- Line e9a22d10-c169-4cb9-b823-11c73169328c/LConn2 -- Line 1716516389/RConn2 -- Line 89d3125f-fc75-4299-8889-5174924ee4ad/LConn2
  Line c3bd0772-1c61-4059-90cf-b754e0a17fa2/LConn3 -- Line e9a22d10-c169-4cb9-b823-11c73169328c/LConn3 -- Line 1716516389/RConn3 -- Line 89d3125f-fc75-4299-8889-5174924ee4ad/LConn3
  Line 1e7def22-dd71-47a8-aeb6-b820dd984e65/LConn1 -- Line 29ecd01e-d271-4388-90e1-f3eea1c5d3e5/LConn1 -- Line 687c6ab8-3be1-480c-a391-1a50fba3e886/RConn1
  Line 1e7def22-dd71-47a8-aeb6-b820dd984e65/LConn2 -- Line 29ecd01e-d271-4388-90e1-f3eea1c5d3e5/LConn2 -- Line 687c6ab8-3be1-480c-a391-1a50fba3e886/RConn2
  Line 1e7def22-dd71-47a8-aeb6-b820dd984e65/LConn3 -- Line 29ecd01e-d271-4388-90e1-f3eea1c5d3e5/LConn3 -- Line 687c6ab8-3be1-480c-a391-1a50fba3e886/RConn3
  Line 867f1459-8b81-4976-9bab-74549e53d0e3/LConn1 -- Line 285053675/LConn1 -- Line 458366992/RConn1
  Line 867f1459-8b81-4976-9bab-74549e53d0e3/LConn2 -- Line 285053675/LConn2 -- Line 458366992/RConn2
  Line 867f1459-8b81-4976-9bab-74549e53d0e3/LConn3 -- Line 285053675/LConn3 -- Line 458366992/RConn3
  Line/RConn1 -- 8072826a-23ba-4558-b3cc-d08b3134df5b/LConn1
  Line/RConn2 -- 8072826a-23ba-4558-b3cc-d08b3134df5b/LConn2
  Line/RConn3 -- 8072826a-23ba-4558-b3cc-d08b3134df5b/LConn3
  трансформатор Т-2_ЗТП-377/LConn1 -- Line 011b7135-821d-4d95-bc11-3e72dddd44ae/RConn1
  трансформатор Т-2_ЗТП-377/LConn2 -- Line 011b7135-821d-4d95-bc11-3e72dddd44ae/RConn2
  трансформатор Т-2_ЗТП-377/LConn3 -- Line 011b7135-821d-4d95-bc11-3e72dddd44ae/RConn3
  Line f1c9c718-c36b-41ce-b023-8d4f642f603e/LConn1 -- Line c3bd0772-1c61-4059-90cf-b754e0a17fa2/RConn1
  Line f1c9c718-c36b-41ce-b023-8d4f642f603e/LConn2 -- Line c3bd0772-1c61-4059-90cf-b754e0a17fa2/RConn2
  Line f1c9c718-c36b-41ce-b023-8d4f642f603e/LConn3 -- Line c3bd0772-1c61-4059-90cf-b754e0a17fa2/RConn3
  Line 458366992/LConn1 -- 8072826a-23ba-4558-b3cc-d08b3134df5b/RConn1
  Line 458366992/LConn2 -- 8072826a-23ba-4558-b3cc-d08b3134df5b/RConn2
  Line 458366992/LConn3 -- 8072826a-23ba-4558-b3cc-d08b3134df5b/RConn3
  Line d60e7ae4-54f0-4b2e-a601-9678671982ab/LConn1 -- Line -379141262/LConn1 -- Line 2120786381/RConn1
  Line d60e7ae4-54f0-4b2e-a601-9678671982ab/LConn2 -- Line -379141262/LConn2 -- Line 2120786381/RConn2
  Line d60e7ae4-54f0-4b2e-a601-9678671982ab/LConn3 -- Line -379141262/LConn3 -- Line 2120786381/RConn3
  трансформатор Т-2_ЗТП-1073/LConn1 -- Line 29ecd01e-d271-4388-90e1-f3eea1c5d3e5/RConn1
  трансформатор Т-2_ЗТП-1073/LConn2 -- Line 29ecd01e-d271-4388-90e1-f3eea1c5d3e5/RConn2
  трансформатор Т-2_ЗТП-1073/LConn3 -- Line 29ecd01e-d271-4388-90e1-f3eea1c5d3e5/RConn3
  Line 5fe16979-df1f-4ffc-8e8c-eea579151a4f/LConn1 -- Line 566348843/LConn1 -- Line 1362246896/RConn1
  Line 5fe16979-df1f-4ffc-8e8c-eea579151a4f/LConn2 -- Line 566348843/LConn2 -- Line 1362246896/RConn2
  Line 5fe16979-df1f-4ffc-8e8c-eea579151a4f/LConn3 -- Line 566348843/LConn3 -- Line 1362246896/RConn3
  трансформатор Т-1_ЗТП-377/LConn1 -- Line 2b3928e6-1e74-4724-a381-14e26628662e/RConn1
  трансформатор Т-1_ЗТП-377/LConn2 -- Line 2b3928e6-1e74-4724-a381-14e26628662e/RConn2
  трансформатор Т-1_ЗТП-377/LConn3 -- Line 2b3928e6-1e74-4724-a381-14e26628662e/RConn3
